simulink model "Hopper_3DOF_v1_7"  (R2025a)
settings: Solver=VariableStepAuto  StartTime=0.0  StopTime=100  RelTol=1e-3
values from neighbouring files (symbols this model uses):
  g = 9.80665    [vehicle_info.m]
  I = [ I_xx, 0,     0 ... (first row only)    [vehicle_info.m]
  m0 = 48    [vehicle_info.m]
  mdot = 0    [vehicle_info.m]
  mt = 114    [vehicle_info.m]
libraries: slpidlib x3, aerolibanim x2, aerolibobsolete x1, simulink_extras x1
settings Model: Creator=vip  LastModifiedBy=asing

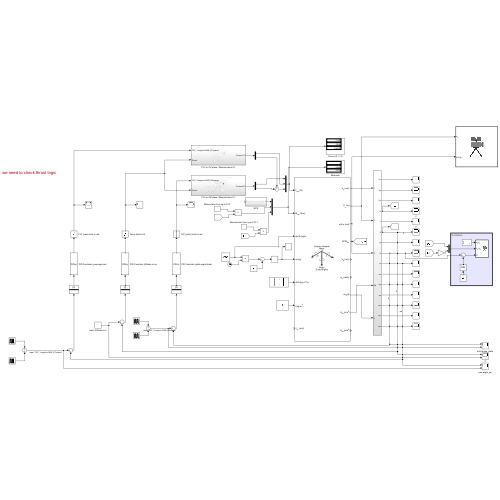
[thumbnail: Simulink's stored preview of the top-level diagram]
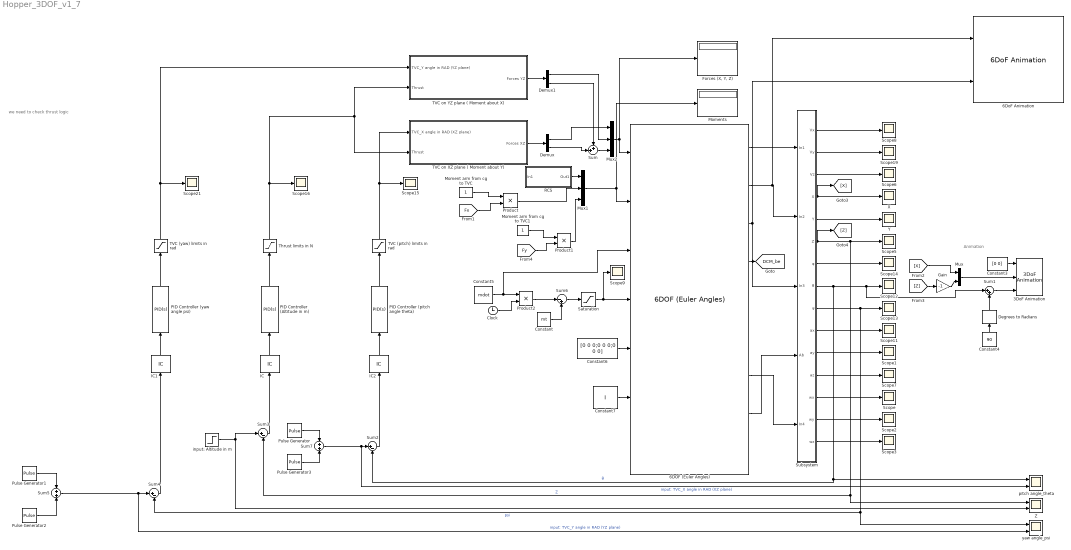
== system Hopper_3DOF_v1_7 ==
  note: we need to check thrust logic
  note: Animation
  3DoF Animation : aerolibanim/3DoF Animation  u1=[-5 5 -10 10 -250 0]  u2=0.05  u3=0.1  u5=Fly alongside  u6=[10 10 0]  u7=70  u8=off
  6DOF (Euler Angles) : aerolibobsolete/6DOF (Euler Angles)  units=Metric (MKS)  mtype=Custom Variable  rep=Euler Angles  xme_0=[0 0 0]  Vm_0=[0 0 0]  eul_0=[0 0 0]  pm_0=[0 0 0]  mass_0=4  mass_e=0.5  mass_f=2.0  inertia=[43 0 0 ; 0 43 0; 0 0 43]  inertia_e=eye(3)  inertia_f=2*eye(3)  k_quat=1.0  vre_flag=on  abi_flag=on  aMode=0  xme_statename=''  Vm_statename=''  eul_statename=''  quat_statename=''  pm_statename=''  mass_statename=''
  6DoF Animation : aerolibanim/6DoF Animation  u1=[-5 5 -10 10 -250 0]  u2=0.05  u3=5  u4=[4 0 -5]  u5=Fly alongside  u6=[10 10 0]  u7=70  u8=on
  Clock : Clock
  Constant : Constant  Value=mt
  Constant3 : Constant  Value=[0 0]
  Constant4 : Constant  Value=90
  Constant5 : Constant  Value=mdot
  Constant6 : Constant  Value=[0 0 0;0 0 0;0 0 0]
  Constant7 : Constant  Value=I
  Degrees to Radians : simulink_extras/Transformations/Degrees to Radians
  Demux : Demux  Outputs=2
  Demux1 : Demux  Outputs=2
  "Forces (X, Y, Z)" : Display
  Gain : Gain  Gain=-1
  IC : InitialCondition  Value=0
  IC1 : InitialCondition  Value=0
  IC2 : InitialCondition  Value=0
  Moment arm from cg to TVC : Constant
  Moment arm from cg to TVC1 : Constant
  Moments : Display
  Mux : Mux  Inputs=2
  Mux1 : Mux  Inputs=3
  Mux2 : Mux  Inputs=3
  PID Controller (Altitude in m) : slpidlib/PID Controller  Controller=PID  Form=Parallel  TimeDomain=Continuous-time  UseExternalTs=off  SampleTime=-1  IntegratorMethod=Forward Euler  FilterMethod=Forward Euler  ControllerParametersSource=internal  P=9.5  I=0.8  UseKiTs=off  D=12  UseExternalDerivativeSource=off  N=50  UseFilter=on  TunerSelectOption=Transfer Function Based (PID Tuner App)  InitialConditionSource=internal  InitialConditionForIntegrator=0  InitialConditionForFilter=0  DifferentiatorICPrevScaledInput=0  ExternalReset=none  TrackingMode=off  Kt=1  LimitOutput=off  SatLimitsSource=internal  UpperSaturationLimit=800  LowerSaturationLimit=0  LinearizeAsGain=off  AntiWindupMode=clamping  Kb=1  LimitIntegrator=off  UpperIntegratorSaturationLimit=1000  LowerIntegratorSaturationLimit=0  POutMin=[]  POutMax=[]  IOutMin=[]  IOutMax=[]  DOutMin=[]  DOutMax=[]  NOutMin=[]  NOutMax=[]  SumOutMin=[]  SumOutMax=[]  SaturationOutMin=[]  SaturationOutMax=[]  PParamMin=[]  PParamMax=[]  IParamMin=[]  IParamMax=[]  DParamMin=[]  DParamMax=[]  NParamMin=[]  NParamMax=[]  KbParamMin=[]  KbParamMax=[]  KtParamMin=[]  KtParamMax=[]  KbOutMin=[]  KbOutMax=[]  KtOutMin=[]  KtOutMax=[]  IntegratorOutMin=[]  IntegratorOutMax=[]  FilterOutMin=[]  FilterOutMax=[]  SumI1OutMin=[]  SumI1OutMax=[]  SumI2OutMin=[]  SumI2OutMax=[]  SumI3OutMin=[]  SumI3OutMax=[]  SumI4OutMin=[]  SumI4OutMax=[]  SumDOutMin=[]  SumDOutMax=[]  DifferentiatorOutMin=[]  DifferentiatorOutMax=[]  FilterDiffOutCoefMin=[]  FilterDiffOutCoefMax=[]  ReciprocalOutMin=[]  ReciprocalOutMax=[]  SumDenOutMin=[]  SumDenOutMax=[]  SumNumOutMin=[]  SumNumOutMax=[]  DivideOutMin=[]  DivideOutMax=[]  UdiffTsProdOutMin=[]  UdiffTsProdOutMax=[]  NTsProdOutMin=[]  NTsProdOutMax=[]  UintegralTsProdOutMin=[]  UintegralTsProdOutMax=[]  UngainTsProdOutMin=[]  UngainTsProdOutMax=[]  ClampingZeroOutDataTypeStr=Inherit: Inherit via back propagation  ClampingZeroOutMin=[]  ClampingZeroOutMax=[]  FilterDenConstantOutDataTypeStr=Inherit: Inherit via back propagation  FilterDenConstantOutMin=[]  FilterDenConstantOutMax=[]  PCopyOutDataTypeStr=Inherit: Inherit via back propagation  PCopyOutMin=[]  PCopyOutMax=[]  NCopyOutDataTypeStr=Inherit: Inherit via back propagation  NCopyOutMin=[]  NCopyOutMax=[]  IntegratorContinuousStateAttributes=''  IntegratorStateMustResolveToSignalObject=off  IntegratorRTWStateStorageClass=Auto  FilterContinuousStateAttributes=''  FilterStateMustResolveToSignalObject=off  FilterRTWStateStorageClass=Auto  ParallelPVariant=InternalParameters  IdealPVariant=Disabled  IVariant=InternalParameters  DVariant=InternalParameters  IntegratorVariant=Continuous  SatVariant=Disabled  AWVariant=Passthrough  PCopyVariant=Disabled  TRVariant=Disabled  FdbkBlocksVariant=Forward  IdealPFdbkVariant=Disabled  SatFdbkVariant=Disabled  DerivativeFilterVariant=ContFilter  NVariant=InternalParameters  NCopyVariant=Disabled  FilterICVariant=InternalICsFilter  IntegratorICVariant=InternalICs  ExternalResetVariant=Disabled  TRSumVariant=Passthrough  SumFdbkVariant=Disabled  SumVariant=Sum_PID  TsampFilterVariant=InternalTs  TsampNgainVariant=Passthrough  TsampIntegralVariant=Disabled_SignalSpec  ExternalSaturationOutDataTypeStr=Inherit: Same as second input  DerivativeSourceVariant=ErrorSignal  PreIntVariant=InternalPreInt
  PID Controller (pitch angle theta) : slpidlib/PID Controller  Controller=PID  Form=Parallel  TimeDomain=Continuous-time  UseExternalTs=off  SampleTime=-1  IntegratorMethod=Forward Euler  FilterMethod=Forward Euler  ControllerParametersSource=internal  P=16.7296251808198  I=1.49026602502535  UseKiTs=off  D=46.0228594879273  UseExternalDerivativeSource=off  N=15  UseFilter=on  TunerSelectOption=Transfer Function Based (PID Tuner App)  InitialConditionSource=internal  InitialConditionForIntegrator=0  InitialConditionForFilter=0  DifferentiatorICPrevScaledInput=0  ExternalReset=none  TrackingMode=off  Kt=1  LimitOutput=off  SatLimitsSource=internal  UpperSaturationLimit=0.25  LowerSaturationLimit=-0.25  LinearizeAsGain=on  AntiWindupMode=clamping  Kb=1  LimitIntegrator=off  UpperIntegratorSaturationLimit=300  LowerIntegratorSaturationLimit=0  POutMin=[]  POutMax=[]  IOutMin=[]  IOutMax=[]  DOutMin=[]  DOutMax=[]  NOutMin=[]  NOutMax=[]  SumOutMin=[]  SumOutMax=[]  SaturationOutMin=[]  SaturationOutMax=[]  PParamMin=[]  PParamMax=[]  IParamMin=[]  IParamMax=[]  DParamMin=[]  DParamMax=[]  NParamMin=[]  NParamMax=[]  KbParamMin=[]  KbParamMax=[]  KtParamMin=[]  KtParamMax=[]  KbOutMin=[]  KbOutMax=[]  KtOutMin=[]  KtOutMax=[]  IntegratorOutMin=[]  IntegratorOutMax=[]  FilterOutMin=[]  FilterOutMax=[]  SumI1OutMin=[]  SumI1OutMax=[]  SumI2OutMin=[]  SumI2OutMax=[]  SumI3OutMin=[]  SumI3OutMax=[]  SumI4OutMin=[]  SumI4OutMax=[]  SumDOutMin=[]  SumDOutMax=[]  DifferentiatorOutMin=[]  DifferentiatorOutMax=[]  FilterDiffOutCoefMin=[]  FilterDiffOutCoefMax=[]  ReciprocalOutMin=[]  ReciprocalOutMax=[]  SumDenOutMin=[]  SumDenOutMax=[]  SumNumOutMin=[]  SumNumOutMax=[]  DivideOutMin=[]  DivideOutMax=[]  UdiffTsProdOutMin=[]  UdiffTsProdOutMax=[]  NTsProdOutMin=[]  NTsProdOutMax=[]  UintegralTsProdOutMin=[]  UintegralTsProdOutMax=[]  UngainTsProdOutMin=[]  UngainTsProdOutMax=[]  ClampingZeroOutDataTypeStr=Inherit: Inherit via back propagation  ClampingZeroOutMin=[]  ClampingZeroOutMax=[]  FilterDenConstantOutDataTypeStr=Inherit: Inherit via back propagation  FilterDenConstantOutMin=[]  FilterDenConstantOutMax=[]  PCopyOutDataTypeStr=Inherit: Inherit via back propagation  PCopyOutMin=[]  PCopyOutMax=[]  NCopyOutDataTypeStr=Inherit: Inherit via back propagation  NCopyOutMin=[]  NCopyOutMax=[]  IntegratorContinuousStateAttributes=''  IntegratorStateMustResolveToSignalObject=off  IntegratorRTWStateStorageClass=Auto  FilterContinuousStateAttributes=''  FilterStateMustResolveToSignalObject=off  FilterRTWStateStorageClass=Auto  ParallelPVariant=InternalParameters  IdealPVariant=Disabled  IVariant=InternalParameters  DVariant=InternalParameters  IntegratorVariant=Continuous  SatVariant=Disabled  AWVariant=Passthrough  PCopyVariant=Disabled  TRVariant=Disabled  FdbkBlocksVariant=Forward  IdealPFdbkVariant=Disabled  SatFdbkVariant=Disabled  DerivativeFilterVariant=ContFilter  NVariant=InternalParameters  NCopyVariant=Disabled  FilterICVariant=InternalICsFilter  IntegratorICVariant=InternalICs  ExternalResetVariant=Disabled  TRSumVariant=Passthrough  SumFdbkVariant=Disabled  SumVariant=Sum_PID  TsampFilterVariant=InternalTs  TsampNgainVariant=Passthrough  TsampIntegralVariant=Disabled_SignalSpec  ExternalSaturationOutDataTypeStr=Inherit: Same as second input  DerivativeSourceVariant=ErrorSignal  PreIntVariant=InternalPreInt
  PID Controller (yaw angle psi) : slpidlib/PID Controller  Controller=PID  Form=Parallel  TimeDomain=Continuous-time  UseExternalTs=off  SampleTime=-1  IntegratorMethod=Forward Euler  FilterMethod=Forward Euler  ControllerParametersSource=internal  P=16.7296251808198  I=1.49026602502535  UseKiTs=off  D=46.0228594879273  UseExternalDerivativeSource=off  N=15  UseFilter=on  TunerSelectOption=Transfer Function Based (PID Tuner App)  InitialConditionSource=internal  InitialConditionForIntegrator=0  InitialConditionForFilter=0  DifferentiatorICPrevScaledInput=0  ExternalReset=none  TrackingMode=off  Kt=1  LimitOutput=off  SatLimitsSource=internal  UpperSaturationLimit=0.25  LowerSaturationLimit=-0.25  LinearizeAsGain=on  AntiWindupMode=clamping  Kb=1  LimitIntegrator=off  UpperIntegratorSaturationLimit=300  LowerIntegratorSaturationLimit=0  POutMin=[]  POutMax=[]  IOutMin=[]  IOutMax=[]  DOutMin=[]  DOutMax=[]  NOutMin=[]  NOutMax=[]  SumOutMin=[]  SumOutMax=[]  SaturationOutMin=[]  SaturationOutMax=[]  PParamMin=[]  PParamMax=[]  IParamMin=[]  IParamMax=[]  DParamMin=[]  DParamMax=[]  NParamMin=[]  NParamMax=[]  KbParamMin=[]  KbParamMax=[]  KtParamMin=[]  KtParamMax=[]  KbOutMin=[]  KbOutMax=[]  KtOutMin=[]  KtOutMax=[]  IntegratorOutMin=[]  IntegratorOutMax=[]  FilterOutMin=[]  FilterOutMax=[]  SumI1OutMin=[]  SumI1OutMax=[]  SumI2OutMin=[]  SumI2OutMax=[]  SumI3OutMin=[]  SumI3OutMax=[]  SumI4OutMin=[]  SumI4OutMax=[]  SumDOutMin=[]  SumDOutMax=[]  DifferentiatorOutMin=[]  DifferentiatorOutMax=[]  FilterDiffOutCoefMin=[]  FilterDiffOutCoefMax=[]  ReciprocalOutMin=[]  ReciprocalOutMax=[]  SumDenOutMin=[]  SumDenOutMax=[]  SumNumOutMin=[]  SumNumOutMax=[]  DivideOutMin=[]  DivideOutMax=[]  UdiffTsProdOutMin=[]  UdiffTsProdOutMax=[]  NTsProdOutMin=[]  NTsProdOutMax=[]  UintegralTsProdOutMin=[]  UintegralTsProdOutMax=[]  UngainTsProdOutMin=[]  UngainTsProdOutMax=[]  ClampingZeroOutDataTypeStr=Inherit: Inherit via back propagation  ClampingZeroOutMin=[]  ClampingZeroOutMax=[]  FilterDenConstantOutDataTypeStr=Inherit: Inherit via back propagation  FilterDenConstantOutMin=[]  FilterDenConstantOutMax=[]  PCopyOutDataTypeStr=Inherit: Inherit via back propagation  PCopyOutMin=[]  PCopyOutMax=[]  NCopyOutDataTypeStr=Inherit: Inherit via back propagation  NCopyOutMin=[]  NCopyOutMax=[]  IntegratorContinuousStateAttributes=''  IntegratorStateMustResolveToSignalObject=off  IntegratorRTWStateStorageClass=Auto  FilterContinuousStateAttributes=''  FilterStateMustResolveToSignalObject=off  FilterRTWStateStorageClass=Auto  ParallelPVariant=InternalParameters  IdealPVariant=Disabled  IVariant=InternalParameters  DVariant=InternalParameters  IntegratorVariant=Continuous  SatVariant=Disabled  AWVariant=Passthrough  PCopyVariant=Disabled  TRVariant=Disabled  FdbkBlocksVariant=Forward  IdealPFdbkVariant=Disabled  SatFdbkVariant=Disabled  DerivativeFilterVariant=ContFilter  NVariant=InternalParameters  NCopyVariant=Disabled  FilterICVariant=InternalICsFilter  IntegratorICVariant=InternalICs  ExternalResetVariant=Disabled  TRSumVariant=Passthrough  SumFdbkVariant=Disabled  SumVariant=Sum_PID  TsampFilterVariant=InternalTs  TsampNgainVariant=Passthrough  TsampIntegralVariant=Disabled_SignalSpec  ExternalSaturationOutDataTypeStr=Inherit: Same as second input  DerivativeSourceVariant=ErrorSignal  PreIntVariant=InternalPreInt
  Product : Product
  Product1 : Product
  Product2 : Product
  Pulse Generator : DiscretePulseGenerator  PulseType=Time based  Amplitude=0.1  Period=100  PulseWidth=10  PhaseDelay=10
  Pulse Generator1 : DiscretePulseGenerator  PulseType=Time based  Amplitude=-0.1  Period=100  PulseWidth=10  PhaseDelay=20
  Pulse Generator2 : DiscretePulseGenerator  PulseType=Time based  Amplitude=0.1  Period=100  PulseWidth=10  PhaseDelay=10
  Pulse Generator3 : DiscretePulseGenerator  PulseType=Time based  Amplitude=-0.1  Period=100  PulseWidth=10  PhaseDelay=20
  RCS : Subsystem
  Saturation : Saturate  UpperLimit=mt  LowerLimit=m0
  Scope{,1..3,5..9,11..16,19,21} (17 alike) : Scope
      Scope settings: ActiveDisplayYMinimum=-1  ActiveDisplayYMaximum=1  DataLoggingVariableName=ScopeData10
      Scope1 settings: ActiveDisplayYMinimum=-1  ActiveDisplayYMaximum=1
      Scope11 settings: ActiveDisplayYMinimum=-1  ActiveDisplayYMaximum=1  DataLoggingVariableName=ScopeData6
      Scope12 settings: ActiveDisplayYMinimum=-1  ActiveDisplayYMaximum=1  DataLoggingVariableName=ScopeData7
      Scope13 settings: ActiveDisplayYMinimum=-1  ActiveDisplayYMaximum=1  DataLoggingVariableName=ScopeData8
      Scope14 settings: ActiveDisplayYMinimum=-0.40362  ActiveDisplayYMaximum=0.917  DataLoggingVariableName=ScopeData9
      Scope15 settings: ActiveDisplayYMinimum=-0.3125  ActiveDisplayYMaximum=0.3125  DataLoggingVariableName=ScopeData13
      Scope16 settings: ActiveDisplayYMinimum=-166.25  ActiveDisplayYMaximum=1496.25  DataLoggingVariableName=ScopeData17
      Scope19 settings: ActiveDisplayYMinimum=-1  ActiveDisplayYMaximum=1  DataLoggingVariableName=ScopeData16
      Scope2 settings: ActiveDisplayYMinimum=-0.01484  ActiveDisplayYMaximum=0.12541  DataLoggingVariableName=ScopeData11
      Scope21 settings: ActiveDisplayYMinimum=-0.3125  ActiveDisplayYMaximum=0.3125  DataLoggingVariableName=ScopeData4
      Scope3 settings: ActiveDisplayYMinimum=-1  ActiveDisplayYMaximum=1  DataLoggingVariableName=ScopeData12
      Scope5 settings: ActiveDisplayYMinimum=-6.33646  ActiveDisplayYMaximum=57.02812
      Scope6 settings: ActiveDisplayYMinimum=-56.08961  ActiveDisplayYMaximum=504.80653  DataLoggingVariableName=ScopeData2
      Scope7 settings: ActiveDisplayYMinimum=-1  ActiveDisplayYMaximum=1  DataLoggingVariableName=ScopeData3
      Scope8 settings: ActiveDisplayYMinimum=-1  ActiveDisplayYMaximum=1  DataLoggingVariableName=ScopeData4
      Scope9 settings: ActiveDisplayYMinimum=45  ActiveDisplayYMaximum=75  DataLoggingVariableName=ScopeData2
  Subsystem : Subsystem
  Sum : Sum  Inputs=++|
  Sum1 : Sum  Inputs=|++
  Sum2 : Sum  Inputs=|+-
  Sum3 : Sum  Inputs=|+-
  Sum4 : Sum  Inputs=|+-
  Sum5 : Sum  Inputs=+|+
  Sum6 : Sum  Inputs=|-+
  Sum7 : Sum  Inputs=+|+
  TVC (pitch) limits in rad : Saturate  UpperLimit=0.25  LowerLimit=-0.25
  TVC (yaw) limits in rad : Saturate  UpperLimit=0.25  LowerLimit=-0.25
  TVC on XZ plane ( Moment about Y) : Subsystem
  TVC on YZ plane ( Moment about X) : Subsystem
  Thrust limits in N : Saturate  UpperLimit=1330  LowerLimit=0
  X : Scope
      settings: ActiveDisplayYMinimum=-6.33797  ActiveDisplayYMaximum=42.67544  DataLoggingVariableName=ScopeData5
  Y : Scope
      settings: ActiveDisplayYMinimum=-0.22309  ActiveDisplayYMaximum=1.9929  DataLoggingVariableName=ScopeData20
  Z : Scope  NumInputPorts=2
      settings: ActiveDisplayYMinimum=-12.5  ActiveDisplayYMaximum=112.5  DataLoggingVariableName=ScopeData15
  input: Altitude in m : Step  Time=0  After=100  SampleTime=0
  pitch angle_theta : Scope  NumInputPorts=2
      settings: ActiveDisplayYMinimum=-0.15668346365265828  ActiveDisplayYMaximum=0.13800142038412488
  yaw angle_psi : Scope  NumInputPorts=2
      settings: ActiveDisplayYMinimum=-0.14004553821670884  ActiveDisplayYMaximum=0.13319742393242368  DataLoggingVariableName=ScopeData3
  tag scope: DCM_be=global
  wires:
  Constant6/1 -> 6DOF (Euler Angles)/5
  Mux1/1 -> Moments/1, 6DOF (Euler Angles)/2
  Constant5/1 -> 6DOF (Euler Angles)/3, Product2/1
  Product/1 -> Mux1/2
  Moment arm from cg to TVC/1 -> Product/1
  [Fx] -> Product/2
  Product1/1 -> Mux1/3
  RCS/1(Out1) -> Mux1/1
  Constant7/1 -> 6DOF (Euler Angles)/6
  6DOF (Euler Angles)/4 -> [DCM_be]
  Constant3/1 -> 3DoF Animation/1
  Mux/1 -> 3DoF Animation/2
  Subsystem/4(X) -> [X], X/1
  6DOF (Euler Angles)/1 -> Subsystem/1(In1)
  6DOF (Euler Angles)/2 -> 6DoF Animation/1, Subsystem/2(In2)
  6DOF (Euler Angles)/3 -> Subsystem/3(In3), 6DoF Animation/2
  6DOF (Euler Angles)/7 -> Subsystem/5(In4)
  Subsystem/1(Vx) -> Scope8/1
  Subsystem/2(Vy) -> Scope19/1
  Subsystem/3(Vz) -> Scope6/1
  Subsystem/5(Y) -> Y/1
  Subsystem/7(φ) -> Scope14/1
  Subsystem/10(ax) -> Scope11/1
  Subsystem/11(ay) -> Scope1/1
  Subsystem/12(az) -> Scope7/1
  6DOF (Euler Angles)/8 -> Subsystem/4(Ab)
  Subsystem/13(wx) -> Scope/1
  Subsystem/14(wy) -> Scope2/1
  Subsystem/15(wz) -> Scope3/1
  [X] -> Mux/1
  [Z] -> Gain/1
  PID Controller (Altitude in m)/1 -> Thrust limits in N/1
  Moment arm from cg to TVC1/1 -> Product1/1
  [Fy] -> Product1/2
  TVC on XZ plane ( Moment about Y)/1(Forces XZ) -> Demux/1
  TVC on YZ plane ( Moment about X)/1(Forces YZ) -> Demux1/1
  Mux2/1 -> "Forces (X, Y, Z)"/1, 6DOF (Euler Angles)/1
  Demux/1 -> Mux2/1
  Demux1/1 -> Mux2/2
  Sum/1 -> Mux2/3
  Demux1/2 -> Sum/1
  Demux/2 -> Sum/2
  Sum2/1 -> IC2/1
  Subsystem/8(θ) -> Sum2/2, pitch angle_theta/1, Sum1/1, Scope12/1  "θ"
  PID Controller (pitch angle theta)/1 -> TVC (pitch) limits in rad/1
  Gain/1 -> Mux/2
  Constant4/1 -> Degrees to Radians/1
  Degrees to Radians/1 -> Sum1/2
  Sum1/1 -> 3DoF Animation/3
  input: Altitude in m/1 -> Z/2, Sum3/1
  Sum3/1 -> IC/1
  Subsystem/6(Z) -> [Z], Z/1, Sum3/2, Scope5/1  "Z"
  IC/1 -> PID Controller (Altitude in m)/1
  TVC (pitch) limits in rad/1 -> TVC on XZ plane ( Moment about Y)/1(TVC_X angle in RAD (XZ plane)), Scope15/1
  Subsystem/9(ψ) -> Scope13/1, yaw angle_psi/1, Sum4/2  "psi"
  PID Controller (yaw angle psi)/1 -> TVC (yaw) limits in rad/1
  Sum4/1 -> IC1/1
  IC1/1 -> PID Controller (yaw angle psi)/1
  IC2/1 -> PID Controller (pitch angle theta)/1
  Sum6/1 -> Saturation/1
  Product2/1 -> Sum6/1
  Constant/1 -> Sum6/2
  Clock/1 -> Product2/2
  Saturation/1 -> 6DOF (Euler Angles)/4, Scope9/1
  Thrust limits in N/1 -> Scope16/1, TVC on YZ plane ( Moment about X)/2(Thrust), TVC on XZ plane ( Moment about Y)/2(Thrust)
  TVC (yaw) limits in rad/1 -> TVC on YZ plane ( Moment about X)/1(TVC_Y angle in RAD (YZ plane)), Scope21/1
  Pulse Generator/1 -> Sum7/1
  Pulse Generator1/1 -> Sum5/1
  Pulse Generator2/1 -> Sum5/2
  Sum5/1 -> yaw angle_psi/2, Sum4/1  "input: TVC_Y angle in RAD (YZ plane)"
  Pulse Generator3/1 -> Sum7/2
  Sum7/1 -> pitch angle_theta/2, Sum2/1  "input: TVC_X angle in RAD (XZ plane)"

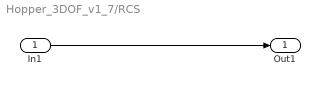
== system Hopper_3DOF_v1_7/RCS ==
  In1 : Inport
  Out1 : Outport
  wires:
  In1/1 -> Out1/1

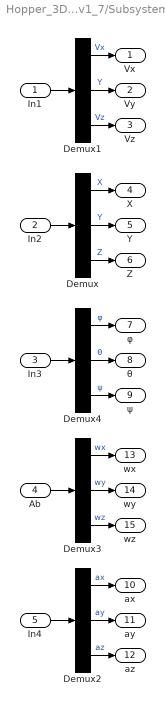
== system Hopper_3DOF_v1_7/Subsystem ==
  In1 : Inport
  In2 : Inport  Port=2
  In3 : Inport  Port=3
  Ab : Inport  Port=4
  In4 : Inport  Port=5
  Demux{,1..4} (5 alike) : Demux  Outputs=3
  Vx : Outport
  Vy : Outport  Port=2
  Vz : Outport  Port=3
  X : Outport  Port=4
  Y : Outport  Port=5
  Z : Outport  Port=6
  φ : Outport  Port=7
  θ : Outport  Port=8
  ψ : Outport  Port=9
  ax : Outport  Port=10
  ay : Outport  Port=11
  az : Outport  Port=12
  wx : Outport  Port=13
  wy : Outport  Port=14
  wz : Outport  Port=15
  wires:
  Demux/3 -> Z/1  "Z"
  Demux4/1 -> φ/1  "φ"
  In2/1 -> Demux/1
  In4/1 -> Demux2/1
  Demux/2 -> Y/1  "Y"
  Demux/1 -> X/1  "X"
  Demux1/3 -> Vz/1  "Vz"
  Demux1/1 -> Vx/1  "Vx"
  Demux4/3 -> ψ/1  "ψ"
  Demux4/2 -> θ/1  "θ"
  Demux2/2 -> ay/1  "ay"
  In1/1 -> Demux1/1
  In3/1 -> Demux4/1
  Demux2/3 -> az/1  "az"
  Demux2/1 -> ax/1  "ax"
  Demux1/2 -> Vy/1  "Y"
  Demux3/1 -> wx/1  "wx"
  Demux3/3 -> wz/1  "wz"
  Demux3/2 -> wy/1  "wy"
  Ab/1 -> Demux3/1

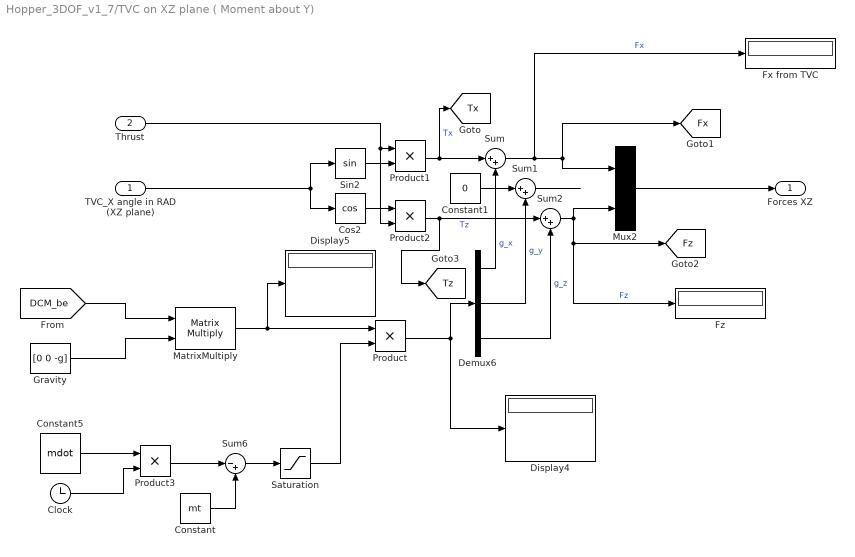
== system Hopper_3DOF_v1_7/TVC on XZ plane ( Moment about Y) ==
  TVC_X angle in RAD (XZ plane) : Inport
  Thrust : Inport  Port=2
  Clock : Clock
  Constant : Constant  Value=mt
  Constant1 : Constant  Value=0
  Constant5 : Constant  Value=mdot
  Cos2 : Trigonometry  Operator=cos
  Demux6 : Demux  Outputs=3
  Display4 : Display
  Display5 : Display
  "Fx from TVC " : Display
  "Fz " : Display
  Gravity : Constant  Value=[0 0 -g]
  MatrixMultiply : Product  Multiplication=Matrix(*)
  Mux2 : Mux  Inputs=2
  Product{,1..3} (4 alike) : Product
  Saturation : Saturate  UpperLimit=mt  LowerLimit=m0
  Sin2 : Trigonometry
  Sum : Sum  Inputs=|++
  Sum1 : Sum  Inputs=|++
  Sum2 : Sum  Inputs=|++
  Sum6 : Sum  Inputs=|-+
  Forces XZ : Outport
  tag scope: Fx=global, Fz=global, Tx=global, Tz=global
  wires:
  Product/1 -> Demux6/1, Display4/1
  Mux2/1 -> Forces XZ/1
  TVC_X angle in RAD (XZ plane)/1 -> Cos2/1, Sin2/1
  Product1/1 -> [Tx], Sum/1  "Tx"
  Sum1/1 -> ?
  Sin2/1 -> Product1/2
  Thrust/1 -> Product2/2, Product1/1
  MatrixMultiply/1 -> Display5/1, Product/1
  Sum/1 -> "Fx from TVC "/1, [Fx], Mux2/1  "Fx"
  Product2/1 -> [Tz], Sum2/1  "Tz"
  Sum2/1 -> "Fz "/1, [Fz], Mux2/2  "Fz"
  Demux6/3 -> Sum2/2  "g_z"
  Constant1/1 -> Sum1/1
  [DCM_be] -> MatrixMultiply/1
  Gravity/1 -> MatrixMultiply/2
  Demux6/2 -> Sum1/2  "g_y"
  Demux6/1 -> Sum/2  "g_x"
  Cos2/1 -> Product2/1
  Saturation/1 -> Product/2
  Product3/1 -> Sum6/1
  Constant5/1 -> Product3/1
  Sum6/1 -> Saturation/1
  Constant/1 -> Sum6/2
  Clock/1 -> Product3/2

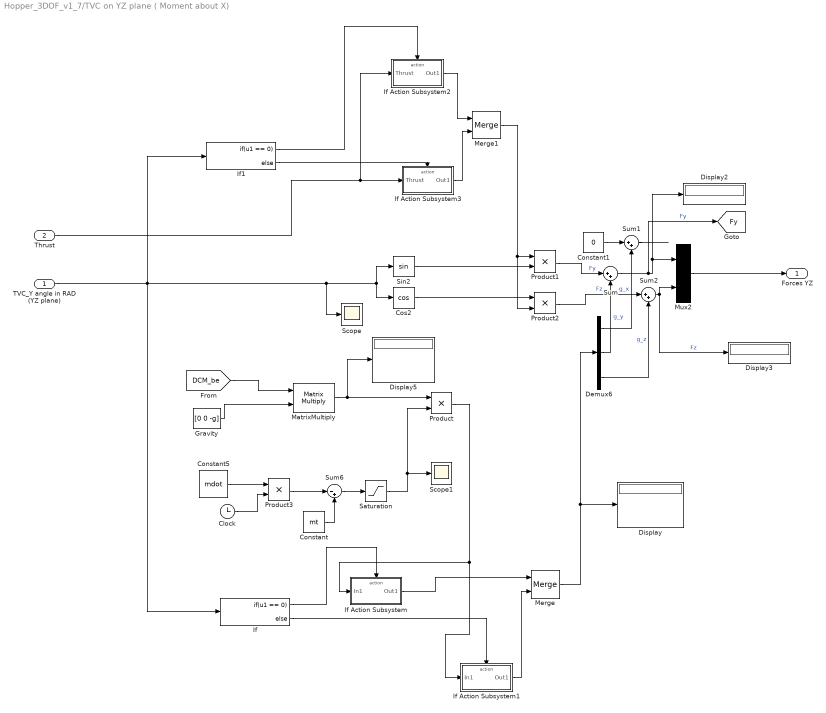
== system Hopper_3DOF_v1_7/TVC on YZ plane ( Moment about X) ==
  TVC_Y angle in RAD (YZ plane) : Inport
  Thrust : Inport  Port=2
  Clock : Clock
  Constant : Constant  Value=mt
  Constant1 : Constant  Value=0
  Constant5 : Constant  Value=mdot
  Cos2 : Trigonometry  Operator=cos
  Demux6 : Demux  Outputs=3
  Display{,2..3,5} (4 alike) : Display
  Gravity : Constant  Value=[0 0 -g]
  If : If  IfExpression=u1 == 0
  If Action Subsystem : Subsystem  TreatAsAtomicUnit=on
  If Action Subsystem1 : Subsystem  TreatAsAtomicUnit=on
  If Action Subsystem2 : Subsystem  TreatAsAtomicUnit=on
  If Action Subsystem3 : Subsystem  TreatAsAtomicUnit=on
  If1 : If  IfExpression=u1 == 0
  MatrixMultiply : Product  Multiplication=Matrix(*)
  Merge : Merge
  Merge1 : Merge
  Mux2 : Mux  Inputs=2
  Product{,1..3} (4 alike) : Product
  Saturation : Saturate  UpperLimit=mt  LowerLimit=m0
  Scope : Scope
      settings: ActiveDisplayYMinimum=-1  ActiveDisplayYMaximum=1  DataLoggingVariableName=ScopeData3
  Scope1 : Scope
      settings: ActiveDisplayYMinimum=45  ActiveDisplayYMaximum=75
  Sin2 : Trigonometry
  Sum : Sum  Inputs=|++
  Sum1 : Sum  Inputs=|++
  Sum2 : Sum  Inputs=|++
  Sum6 : Sum  Inputs=|-+
  Forces YZ : Outport
  tag scope: Fy=global
  wires:
  Cos2/1 -> Product2/1
  Demux6/1 -> Sum1/2  "g_x"
  Demux6/2 -> Sum/2  "g_y"
  Constant1/1 -> Sum1/1
  Demux6/3 -> Sum2/2  "g_z"
  Sum2/1 -> Mux2/2, Display3/1  "Fz"
  Product2/1 -> Sum2/1  "Fz"
  Sum/1 -> [Fy], Mux2/1, Display2/1  "Fy"
  Sin2/1 -> Product1/2
  Sum1/1 -> ?
  Product1/1 -> Sum/1  "Fy"
  TVC_Y angle in RAD (YZ plane)/1 -> If1/1, Scope/1, Sin2/1, Cos2/1, If/1
  Mux2/1 -> Forces YZ/1
  Product/1 -> If Action Subsystem1/1(In1), If Action Subsystem/1(In1)
  MatrixMultiply/1 -> Product/1, Display5/1
  [DCM_be] -> MatrixMultiply/1
  Sum6/1 -> Saturation/1
  Constant/1 -> Sum6/2
  Gravity/1 -> MatrixMultiply/2
  Product3/1 -> Sum6/1
  Saturation/1 -> Product/2, Scope1/1
  Constant5/1 -> Product3/1
  Clock/1 -> Product3/2
  If/1 -> If Action Subsystem/Action
  If Action Subsystem/1(Out1) -> Merge/1
  If Action Subsystem1/1(Out1) -> Merge/2
  If/2 -> If Action Subsystem1/Action
  Merge/1 -> Display/1, Demux6/1
  Thrust/1 -> If Action Subsystem2/1(Thrust), If Action Subsystem3/1(Thrust)
  If Action Subsystem2/1(Out1) -> Merge1/1
  If1/1 -> If Action Subsystem2/Action
  If Action Subsystem3/1(Out1) -> Merge1/2
  If1/2 -> If Action Subsystem3/Action
  Merge1/1 -> Product1/1, Product2/2

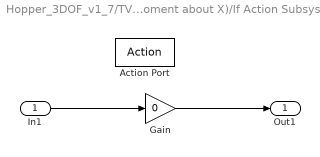
== system Hopper_3DOF_v1_7/TVC on YZ plane ( Moment about X)/If Action Subsystem ==
  In1 : Inport
  Action Port : ActionPort  ActionPortLabel=if(u1 == 0)
  Gain : Gain  Gain=0
  Out1 : Outport
  wires:
  In1/1 -> Gain/1
  Gain/1 -> Out1/1

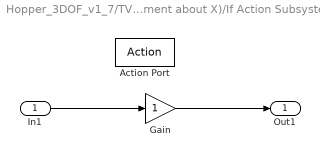
== system Hopper_3DOF_v1_7/TVC on YZ plane ( Moment about X)/If Action Subsystem1 ==
  In1 : Inport
  Action Port : ActionPort  ActionPortLabel=else
  Gain : Gain
  Out1 : Outport
  wires:
  Gain/1 -> Out1/1
  In1/1 -> Gain/1

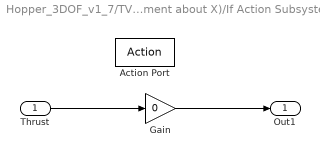
== system Hopper_3DOF_v1_7/TVC on YZ plane ( Moment about X)/If Action Subsystem2 ==
  Thrust : Inport
  Action Port : ActionPort  ActionPortLabel=if(u1 == 0)
  Gain : Gain  Gain=0
  Out1 : Outport
  wires:
  Thrust/1 -> Gain/1
  Gain/1 -> Out1/1

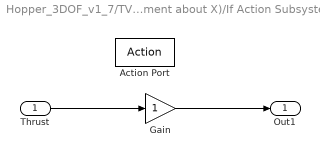
== system Hopper_3DOF_v1_7/TVC on YZ plane ( Moment about X)/If Action Subsystem3 ==
  Thrust : Inport
  Action Port : ActionPort  ActionPortLabel=else
  Gain : Gain
  Out1 : Outport
  wires:
  Gain/1 -> Out1/1
  Thrust/1 -> Gain/1
